simulink model "simulink_05"  (R2023b)
settings: Solver=VariableStepAuto  StartTime=0.0  StopTime=10000  RelTol=1e-3
settings Model: Creator=HP  LastModifiedBy=HP

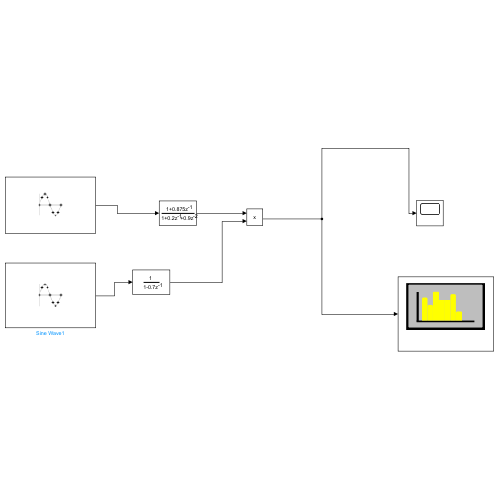
[thumbnail: Simulink's stored preview of the top-level diagram]
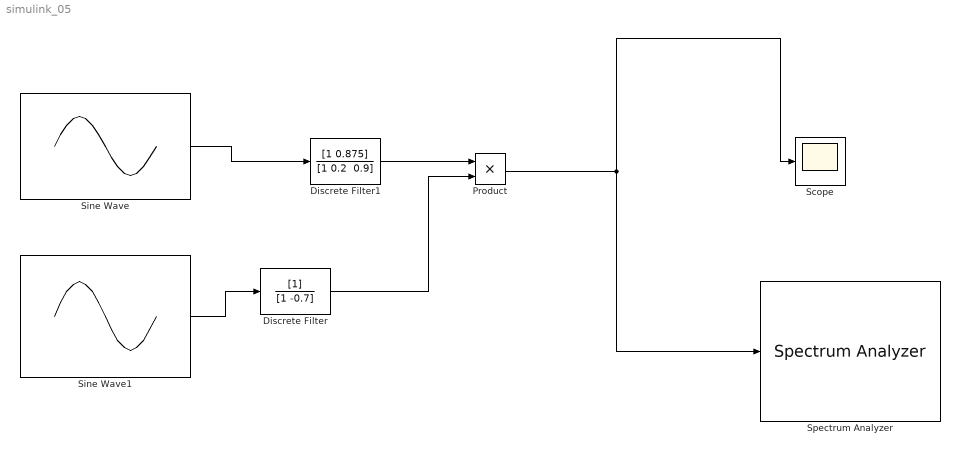
== system simulink_05 ==
  Discrete Filter : DiscreteFilter  Denominator=[1 -0.7]  FilterStructure=Direct form I
  Discrete Filter1 : DiscreteFilter  Numerator=[1 0.875]  Denominator="[1 0.2  0.9]"  FilterStructure=Direct form I
  Product : Product
  Scope : Scope
  Sine Wave : Sin  SineType=Sample based  SampleTime=1
  Sine Wave1 : Sin  SineType=Sample based  SampleTime=1
  Spectrum Analyzer : SpectrumAnalyzer  WindowPosition=[276.000000,58.000000,803.000000,500.000000,]  Visible=on  ScopeFrameLocation=window  Span=1  StartFrequency=-0.5  StopFrequency=0.5  YLimits=[-78.3186322,28.86514057]
  wires:
  Discrete Filter1/1 -> Product/1
  Discrete Filter/1 -> Product/2
  Product/1 -> Scope/1, Spectrum Analyzer/1
  Sine Wave/1 -> Discrete Filter1/1
  Sine Wave1/1 -> Discrete Filter/1
